simulink model "sec_review"  (R2024a)
settings: Solver=VariableStepAuto  StartTime=0.0  StopTime=10.0  RelTol=1e-3
libraries: spsAsynchronousMachinepuUnitsLib x1, spsDCVoltageSourceLib x1, spsUniversalBridgeLib x1, spspowerguiLib x1
settings Model: Creator=vani1  LastModifiedBy=vani1

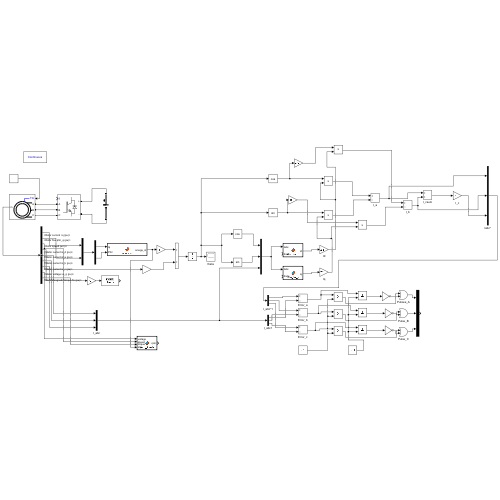
[thumbnail: Simulink's stored preview of the top-level diagram]
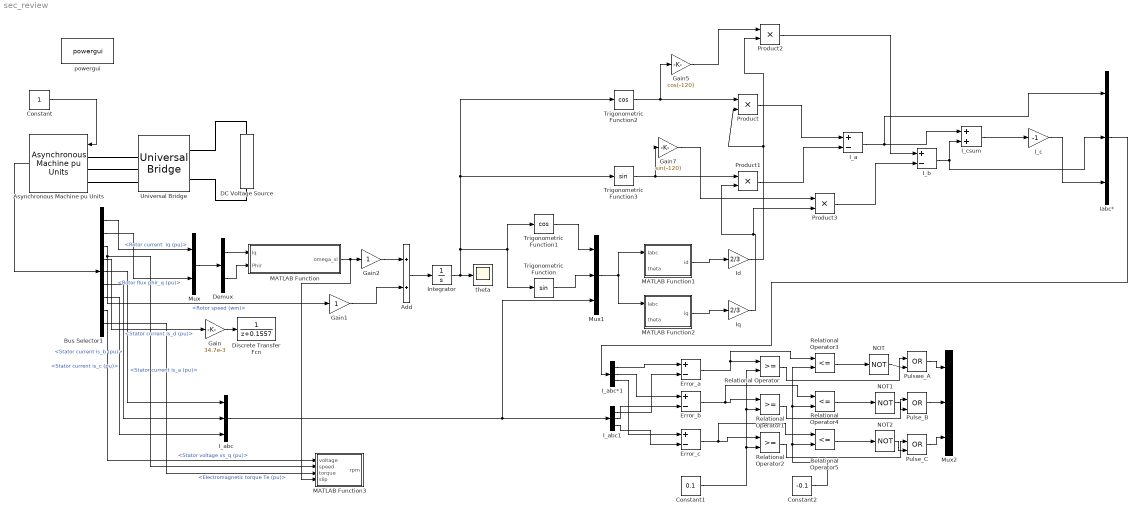
== system sec_review ==
  Add : Sum
  Asynchronous Machine pu Units : spsAsynchronousMachinepuUnitsLib/Asynchronous Machine pu Units  RotorType=Squirrel-cage  PresetModel=No  MechanicalLoad=Torque Tm  ShowDetailedParameters=on  ReferenceFrame=Rotor  Units=pu  MeasurementBus=off  NominalParameters=[3730 460 60]  VoltageRatio=1  Stator=[0.01965 0.0397]  Rotor=[0.01909 0.0397]  Cage1=[0.01909 0.0397]  Cage2=[0.01909 0.0397]  Lm=1.354  Mechanical=[0.09526 0.05479 2]  PolePairs=2  InitialConditions="[ 1,0   0,0,0   0,0,0 ]"  SimulateSaturation=off  Saturation="[0.212,0.4201,0.8125,1.0979,1.4799,2.2457,3.2586,4.5763,6.4763 ;   0.5,0.7,0.9,1,1.1,1.2 ,1.3,1.4,1.5]"  LoadFlowParameters=0  TsPowergui=0  TsBlock=-1  IterativeModel=Trapezoidal non iterative  IterativeDiscreteModel=Trapezoidal non iterative  Pmec=0
      settings: LibrarySourceBlock=|
      | sps_lib/Electrical Machines/Asynchronous Machine
      | pu Units
  Bus Selector1 : BusSelector  OutputSignals="Rotor measurements.Rotor current  iq (pu),Rotor measurements.Rotor flux phir_q (pu),Mechanical.Rotor speed (wm),Stator measurements.Stator current is_d (pu),Stator measurements.Stator current is_a (pu),Stator measurements.Stator current is_b (pu),Stator measurements.Stator current is_c (pu),Stator measurements.Stator voltage vs_q (pu),Mechanical.Electromagnetic torque Te (pu)"
  Constant : Constant  SampleTime=-1
  Constant1 : Constant  Value=0.1
  Constant2 : Constant  Value=-0.1
  DC Voltage Source : spsDCVoltageSourceLib/DC Voltage Source  Amplitude=780  Measurements=Voltage
  Demux : Demux  Outputs=2
  Discrete Transfer Fcn : DiscreteTransferFcn  Denominator=[1 0.1557]
  Error_a : Sum  Inputs=+-
  Error_b : Sum  Inputs=+-
  Error_c : Sum  Inputs=+-
  Gain : Gain  Gain=34.7e-3
  Gain1 : Gain
  Gain2 : Gain
  Gain5 : Gain  Gain=cos(-120)
  Gain7 : Gain  Gain=sin(-120)
  I_a : Sum  Inputs=+-
  I_abc : Mux  Inputs=3
  I_abc*1 : Demux  Outputs=3
  I_abc1 : Demux  Outputs=3
  I_b : Sum  Inputs=+-
  I_c : Gain  Gain=-1
  I_csum : Sum
  Iabc* : Mux  Inputs=3
  Id : Gain  Gain=2/3
  Integrator : Integrator
  Iq : Gain  Gain=2/3
  MATLAB Function : MATLAB Function  TreatAsAtomicUnit=on
  MATLAB Function1 : MATLAB Function  TreatAsAtomicUnit=on
  MATLAB Function2 : MATLAB Function  TreatAsAtomicUnit=on
  MATLAB Function3 : MATLAB Function  TreatAsAtomicUnit=on
  Mux : Mux  Inputs=2
  Mux1 : Mux  Inputs=3
  Mux2 : Mux  Inputs=3
  NOT : Logic  Operator=NOT  IconShape=distinctive  AllPortsSameDT=off  OutDataTypeStr=boolean
  NOT1 : Logic  Operator=NOT  IconShape=distinctive  AllPortsSameDT=off  OutDataTypeStr=boolean
  NOT2 : Logic  Operator=NOT  IconShape=distinctive  AllPortsSameDT=off  OutDataTypeStr=boolean
  Product{,1..3} (4 alike) : Product
  Pulse_B : Logic  Operator=OR  IconShape=distinctive  AllPortsSameDT=off  OutDataTypeStr=boolean
  Pulse_C : Logic  Operator=OR  IconShape=distinctive  AllPortsSameDT=off  OutDataTypeStr=boolean
  Pulswe_A : Logic  Operator=OR  IconShape=distinctive  AllPortsSameDT=off  OutDataTypeStr=boolean
  Relational Operator : RelationalOperator  OutDataTypeStr=boolean  RndMeth=Simplest  InputSameDT=off
  Relational Operator1 : RelationalOperator  OutDataTypeStr=boolean  RndMeth=Simplest  InputSameDT=off
  Relational Operator2 : RelationalOperator  OutDataTypeStr=boolean  RndMeth=Simplest  InputSameDT=off
  Relational Operator3 : RelationalOperator  Operator=<=  OutDataTypeStr=boolean  RndMeth=Simplest  InputSameDT=off
  Relational Operator4 : RelationalOperator  Operator=<=  OutDataTypeStr=boolean  RndMeth=Simplest  InputSameDT=off
  Relational Operator5 : RelationalOperator  Operator=<=  OutDataTypeStr=boolean  RndMeth=Simplest  InputSameDT=off
  Trigonometric Function : Trigonometry
  Trigonometric Function1 : Trigonometry  Operator=cos
  Trigonometric Function2 : Trigonometry  Operator=cos
  Trigonometric Function3 : Trigonometry
  Universal Bridge : spsUniversalBridgeLib/Universal Bridge  Arms=3  SnubberResistance=1e5  SnubberCapacitance=inf  Device=IGBT / Diodes  Ron=1e-3  Lon=0  ForwardVoltages="[  0  0  ]"  ForwardVoltage=0  GTOparameters=[ 10e-6 , 20e-6 ]  IGBTparameters=[ 1e-6 , 2e-6 ]  Measurements=None  Measurements_2=None  converterType=Rectifier
  powergui : spspowerguiLib/powergui  Priority=1  SimulationMode=Continuous  SampleTime=50e-6  frequency=60  Iterations=50  frequencyindice=60  Pbase=100e6  ErrMax=1e-4  UnitsV=kV  UnitsW=MW  buscounter=0  FunctionMessages=off  echomessages=off  EnableUseOfTLC=off  CurrentSourceSwitches=off  DisableSnubberDevices=off  DisableRonSwitches=off  DisableVfSwitches=off  DisplayEquations=off  AutomaticDiscreteSolvers=off  SolverType=Tustin/Backward Euler (TBE)  Interpol=off  ExternalGateDelay=off  methode=off  Ts=100  x0status=blocks  SPID=on  SwTol=0  HookPort=off  NonlinearTolerance=1e-4  nMaxIteration=100  ContinueOnMaxIteration=off  RestoreLinks=warning  ResistiveCurrentMeasurement=off  Frange=[0:2:500]  Ylog=off  Xlog=on  ShowGrid=off  save=off  variable=ZData  structure=0  ZoomFFT=off  StartTime=0.0  cycles=1  DisplayStyle=1  fundamental=60  FreqAxis=off  MaxFrequency=1000  frequencyindicesteady=1  RmsSteady=1  display=off
  theta : Scope
  wires:
  Constant/1 -> Asynchronous Machine pu Units/1
  Gain/1 -> Discrete Transfer Fcn/1
  Add/1 -> Integrator/1
  Asynchronous Machine pu Units/1 -> Bus Selector1/1
  Gain1/1 -> Add/2
  Bus Selector1/2 -> Mux/2  "<Rotor flux phir_q (pu)>"
  Bus Selector1/1 -> Mux/1  "<Rotor current  iq (pu)>"
  Bus Selector1/3 -> MATLAB Function3/2(speed), Gain1/1  "<Rotor speed (wm)>"
  Mux/1 -> Demux/1
  Gain2/1 -> Add/1
  Demux/1 -> MATLAB Function/1(Iq)
  Demux/2 -> MATLAB Function/2(Phir)
  MATLAB Function/1(omega_sl) -> MATLAB Function3/4(slip), Gain2/1
  Bus Selector1/4 -> Gain/1  "<Stator current is_d (pu)>"
  Integrator/1 -> Trigonometric Function2/1, Trigonometric Function3/1, Trigonometric Function/1, Trigonometric Function1/1, theta/1
  Trigonometric Function1/1 -> Mux1/1
  Trigonometric Function/1 -> Mux1/2
  Bus Selector1/5 -> I_abc/1  "<Stator current is_a (pu)>"
  Bus Selector1/6 -> I_abc/2  "<Stator current is_b (pu)>"
  Bus Selector1/7 -> I_abc/3  "<Stator current is_c (pu)>"
  I_abc/1 -> Mux1/3, I_abc1/1
  Mux1/1 -> MATLAB Function2/1(Iabc), MATLAB Function1/1(Iabc)
  MATLAB Function1/1(id) -> Id/1
  MATLAB Function2/1(iq) -> Iq/1
  Product/1 -> I_a/1
  Id/1 -> Product2/2, Product/2
  Iq/1 -> Product3/2, Product1/2
  Product1/1 -> I_a/2
  Trigonometric Function2/1 -> Gain5/1, Product/1
  Trigonometric Function3/1 -> Gain7/1, Product1/1
  Gain5/1 -> Product2/1
  Gain7/1 -> Product3/1
  Product2/1 -> I_b/1
  Product3/1 -> I_b/2
  I_a/1 -> Iabc*/1, I_csum/1
  I_b/1 -> I_csum/2, Iabc*/2
  I_csum/1 -> I_c/1
  I_c/1 -> Iabc*/3
  Iabc*/1 -> I_abc*1/1
  I_abc*1/1 -> Error_a/1
  I_abc1/1 -> Error_a/2
  I_abc*1/2 -> Error_b/1
  I_abc1/2 -> Error_b/2
  I_abc*1/3 -> Error_c/1
  I_abc1/3 -> Error_c/2
  Error_a/1 -> Relational Operator3/1, Relational Operator/1
  Error_b/1 -> Relational Operator4/1, Relational Operator1/1
  Error_c/1 -> Relational Operator5/1, Relational Operator2/1
  Constant1/1 -> Relational Operator2/2, Relational Operator1/2, Relational Operator/2
  Constant2/1 -> Relational Operator5/2, Relational Operator4/2, Relational Operator3/2
  Relational Operator3/1 -> NOT/1
  Relational Operator4/1 -> NOT1/1
  Relational Operator5/1 -> NOT2/1
  Relational Operator/1 -> Pulswe_A/1
  Relational Operator1/1 -> Pulse_B/1
  Relational Operator2/1 -> Pulse_C/1
  NOT/1 -> Pulswe_A/2
  NOT1/1 -> Pulse_B/2
  NOT2/1 -> Pulse_C/2
  Pulswe_A/1 -> Mux2/1
  Pulse_B/1 -> Mux2/2
  Pulse_C/1 -> Mux2/3
  Bus Selector1/8 -> MATLAB Function3/1(voltage)  "<Stator voltage vs_q (pu)>"
  Bus Selector1/9 -> MATLAB Function3/3(torque)  "<Electromagnetic torque Te (pu)>"
  connections:
  Asynchronous Machine pu Units/LConn1 -- Universal Bridge/LConn1
  Asynchronous Machine pu Units/LConn2 -- Universal Bridge/LConn2
  Asynchronous Machine pu Units/LConn3 -- Universal Bridge/LConn3
  Universal Bridge/RConn1 -- DC Voltage Source/RConn1
  Universal Bridge/RConn2 -- DC Voltage Source/LConn1

== matlab function sec_review/MATLAB Function1 ==
  data: Iabc input; id output; theta input
function id = abc_to_d(Iabc, theta)
    % Extract phase currents
    Ia = Iabc(1);
    Ib = Iabc(2);
    Ic = Iabc(3);

    % Compute d-axis current
    id = (2/3) * (Ia * cos(theta) + Ib * cos(theta - 2*pi/3) + Ic * cos(theta + 2*pi/3));
end

== matlab function sec_review/MATLAB Function ==
  data: Iq input; omega_sl output; Phir input
function omega_sl = calc_slip(Iq, Phir)
    omega_sl = (34.7e-3 * Iq) / (Phir * 0.1557 + 1e-3);
end

== matlab function sec_review/MATLAB Function2 ==
  data: Iabc input; iq output; theta input
function iq = abc_to_q(Iabc, theta)
    % Extract phase currents
    Ia = Iabc(1);
    Ib = Iabc(2);
    Ic = Iabc(3);

    % Compute q-axis current
    iq = (2/3) * (Ia * sin(theta) + Ib * sin(theta - 2*pi/3) + Ic * sin(theta + 2*pi/3));
end

== matlab function sec_review/MATLAB Function3 ==
  data: voltage input; rpm output; speed input; torque input; slip input
function rpm = ann_block(voltage, speed, torque, slip)
    rpm = ann_predict(voltage, speed, torque, slip);
end
